simulink model "single_robot_control1"  (R2019b)
settings: Solver=FixedStepAuto  StartTime=0.0  StopTime=40  RelTol=1e-3
settings Model: Creator=sanim  LastModifiedBy=Dell
settings DataIOCC: ReturnWorkspaceOutputs=off
settings DebuggingCC: ArithmeticOperatorsInVariantConditions=warning
settings SFSimCC: CustomCodeUndefinedFunction=UseInterfaceOnly

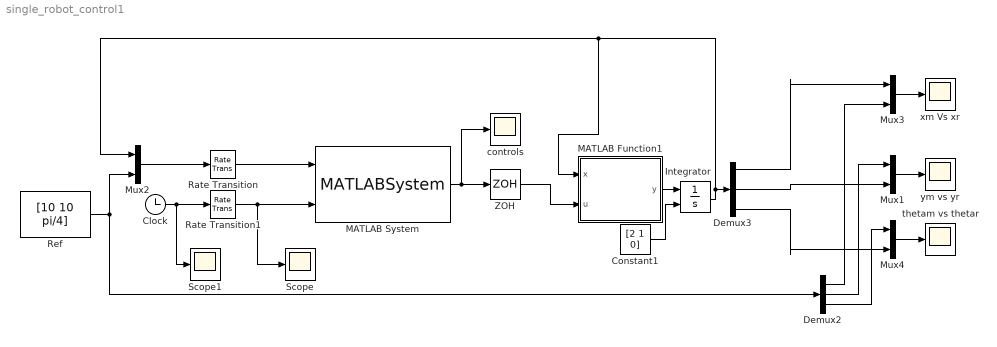
== system single_robot_control1 ==
  Clock : Clock
  Constant1 : Constant  Value=[2 1 0]
  Demux2 : Demux  Outputs=3
  Demux3 : Demux  Outputs=3
  Integrator : Integrator  InitialConditionSource=external  InitialCondition=[1 0]'
  MATLAB Function1 : MATLAB Function  TreatAsAtomicUnit=on
  MATLAB System : MATLABSystem  System=controller  SimulateUsing=Interpreted execution
      mask Type: controller
      mask Display:
      | disp('controller');
      | port_label('input',1,'x');
      | port_label('input',2,'t');
      | port_label('output',1,'u');
  Mux{1..4} (4 alike) : Mux  Inputs=2
  Rate Transition : RateTransition  OutPortSampleTime=0.5
  Rate Transition1 : RateTransition  OutPortSampleTime=0.5
  Ref : Constant  Value=[10 10 pi/4]  VectorParams1D=off
  Scope : Scope
  Scope1 : Scope
  ZOH : ZeroOrderHold  SampleTime=0.5
  controls : Scope
  thetam vs thetar : Scope
  xm Vs xr : Scope
  ym vs yr : Scope
  wires:
  Ref/1 -> Mux2/2, Demux2/1
  Rate Transition/1 -> MATLAB System/1
  MATLAB System/1 -> controls/1, ZOH/1
  Integrator/1 -> MATLAB Function1/1(x), Mux2/1, Demux3/1
  Rate Transition1/1 -> Scope/1, MATLAB System/2
  ZOH/1 -> MATLAB Function1/2(u)
  Clock/1 -> Scope1/1, Rate Transition1/1
  Mux2/1 -> Rate Transition/1
  Demux2/1 -> Mux3/2
  Mux3/1 -> xm Vs xr/1
  Demux2/2 -> Mux1/1
  Mux1/1 -> ym vs yr/1
  Mux4/1 -> thetam vs thetar/1
  Demux2/3 -> Mux4/1
  MATLAB Function1/1(y) -> Integrator/1
  Constant1/1 -> Integrator/2
  Demux3/1 -> Mux3/1
  Demux3/2 -> Mux1/2
  Demux3/3 -> Mux4/2

== matlab function single_robot_control1/MATLAB Function1 ==
  data: x input; y output; u input
function y = rhs(x,u)
%#codegen

y=[u(1)*cos(x(3));u(1)*sin(x(3));u(2)];


end
